simulink model "sine_input"  (R2024a)
settings: Solver=VariableStepAuto  StartTime=0.0  StopTime=10.0  RelTol=1e-3
libraries: slrealtimeiplib x2, dspsrcs4 x1
settings Model: Creator=digital  LastModifiedBy=digital

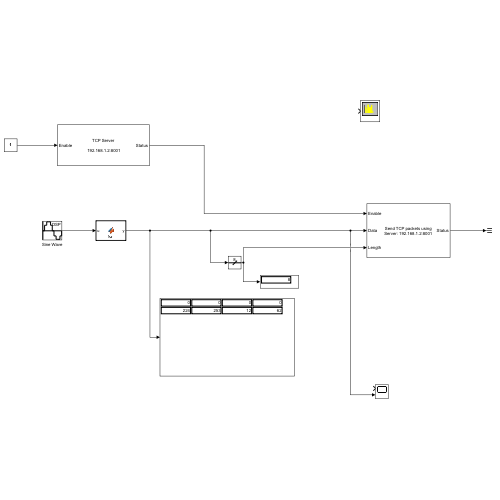
[thumbnail: Simulink's stored preview of the top-level diagram]
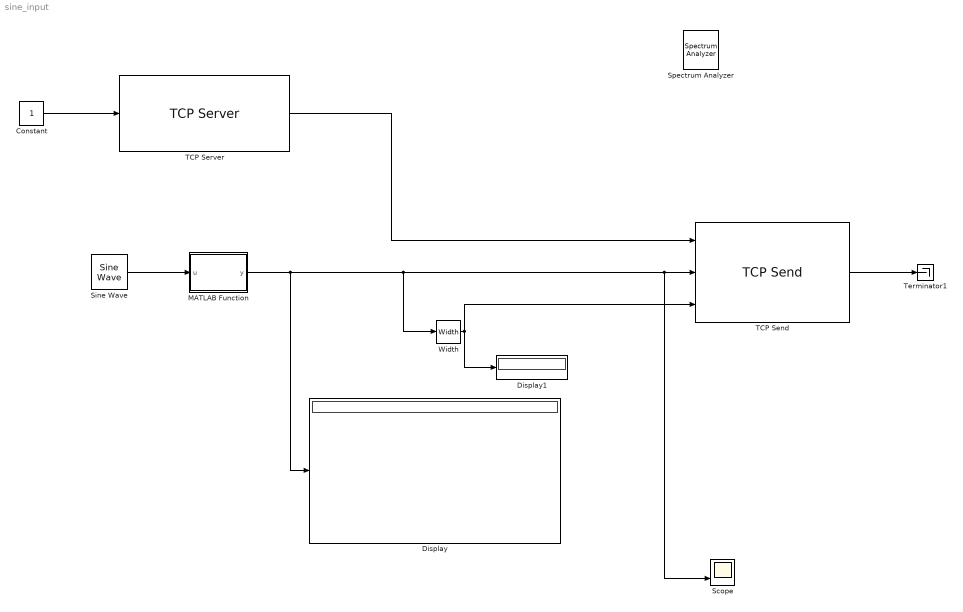
== system sine_input ==
  Constant : Constant
  Display : Display
  Display1 : Display
  MATLAB Function : MATLAB Function  TreatAsAtomicUnit=on
  Scope : Scope  NumInputPorts=2
  Sine Wave : dspsrcs4/Sine Wave  Amplitude=1  Frequency=100  Phase=0  SampleMode=Discrete  OutComplex=Real  CompMethod=Trigonometric fcn  TableSize=Speed  SampleTime=1/1e6  SamplesPerFrame=1  ResetState=Restart at time zero  OutputFrames=off  dataType=double  wordLen=16  udDataType=sfix(16)  fracBitsMode=Best precision  numFracBits=15  OutDataTypeStr=double  LastOutDataTypeStr=double
  Spectrum Analyzer : SpectrumAnalyzer  WindowPosition=[861.000000,533.000000,800.000000,500.000000,]  ScopeFrameLocation=window  Span=2000000  YLimits=[-3603.44492261,-2802.67938425]  SelectedToolstripTab=spectrumAnalyzerToolstrip.estimationTab
  TCP Send : slrealtimeiplib/TCP Send  socketAddPortVal=Server: 192.168.1.2:8001  sampleTime=-1
  TCP Server : slrealtimeiplib/TCP Server  Priority=-1  useHostTargetConn=off  serverAddress=192.168.1.2  serverPort=8001
  Terminator1 : Terminator
  Width : Width
  wires:
  TCP Send/1 -> Terminator1/1
  TCP Server/1 -> TCP Send/1
  Width/1 -> Display1/1, TCP Send/3
  Constant/1 -> TCP Server/1
  MATLAB Function/1(y) -> Width/1, Scope/2, TCP Send/2, Display/1
  Sine Wave/1 -> MATLAB Function/1(u)

== matlab function sine_input/MATLAB Function ==
  data: u input; y output
function y = fcn(u)

y = typecast(u,"uint8");
